simulink model "kinematics_point"  (R2021b)
settings: Solver=VariableStepAuto  StartTime=0.0  StopTime=60  RelTol=1e-10  AbsTol=1e-14
values from neighbouring files (symbols this model uses):
  q0 = [-0.8;0;pi]    [SIM01.m]    (also in SIM02.m = [j 0 the(k)]'; SIM03.m = [-1;0;-pi/2]; SIM04.m = [1 1 k]'; SIM05.m = [2;1;2])
  s0 = [0;0]    [SIM01.m]    (also in SIM02.m; SIM06.m)
settings Model: Creator=PC  LastModifiedBy=PC
settings DataIOCC: SaveFormat=Array
settings DebuggingCC: UnderSpecifiedDimensionMsg=warning

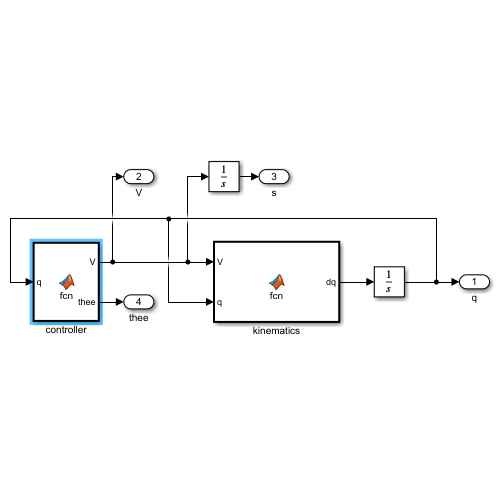
[thumbnail: Simulink's stored preview of the top-level diagram]
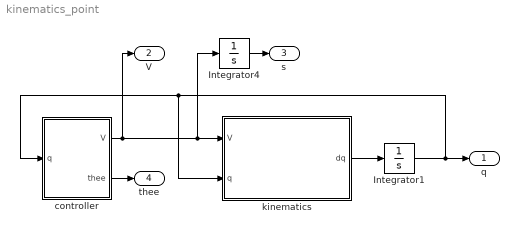
== system kinematics_point ==
  Integrator1 : Integrator  InitialCondition=q0
  Integrator4 : Integrator  InitialCondition=s0
  controller : MATLAB Function  TreatAsAtomicUnit=on
  kinematics : MATLAB Function  TreatAsAtomicUnit=on
  q : Outport
  V : Outport  Port=2
  s : Outport  Port=3
  thee : Outport  Port=4
  wires:
  controller/1(V) -> V/1, kinematics/1(V), Integrator4/1
  Integrator1/1 -> q/1, kinematics/2(q), controller/1(q)
  Integrator4/1 -> s/1
  controller/2(thee) -> thee/1
  kinematics/1(dq) -> Integrator1/1

== matlab function kinematics_point/controller ==
  data: q input size=3*1; V output size=2*1; thee output size=1
function [V,thee]= fcn(q)

the=atan2(sin(q(3)),cos(q(3)));

k1=0.2;k2=0.375;
vm=0.05;wm=0.78;

al=atan2(-q(2),-q(1));    
thee=atan2(sin(al-the),cos(al-the));
d=sqrt(q(2)^2+q(1)^2);
vp=k1*d;
vd=vp*cos(thee*0.5)^2;
v=min(vd,vm);
dal=v*sin(thee)/d;
wd=dal+2*k2*sin(thee*0.5);
w=sign(wd)*min(abs(wd),wm);
V=[v;w];

== matlab function kinematics_point/kinematics ==
  data: V input size=2*1; dq output size=3*1; q input size=3*1
function dq = fcn(V,q)
dq=[ cos(q(3))  0
     sin(q(3))  0
      0         1]*V;
